simulink model "dft_bank_4"  (Simulink 7.8)
settings: Solver=ode45  StartTime=0.0  StopTime=1  RelTol=1e-3
values from neighbouring files (symbols this model uses):
  N = 2    [CFIR_1.m]    (also in TP_fdesign2.m = 128; cic_dezim1.m = ',num2str(N),')']); cic_dezim1_.m = ', num2str(N),' Gain = ',num2str(Hm.gain)]); cic_dezim2.m = ',num2str(N),')']))
  Ts = 1/fs    (= 6.25e-05)    [G722_1.m]    (also in adaptiv_2.m = 0.001; adaptiv_3.m = 0.001; adaptiv_4.m = 0.001; adaptiv_5.m = 0.001)
undefined symbols (not defined in the file or in its folder): Ksub, WN, WNt
libraries: dspsigops x1, dspobslib x1
settings Model: Creator=svenhoffmann  LastModifiedBy=josef  ExtModeAutoUpdateStatusClock=off
settings DataIOCC: SignalLoggingName=sigsOut
settings OptimizationCC: InitFltsAndDblsToZero=on
settings DebuggingCC: SaveWithParameterizedLinksMsg=none  SignalResolutionControl=TryResolveAllWithWarning  SolverPrmCheckMsg=none  MultiTaskDSMMsg=warning  MultiTaskCondExecSysMsg=none  FcnCallInpInsideContextMsg=Use local settings  StrictBusMsg=None
settings HardwareCC: TargetUnknown=on
settings RTWCC: IncludeERTFirstTime=on
settings GRTTargetCC: TargetFcnLib=ansi_tfl_tmw.mat

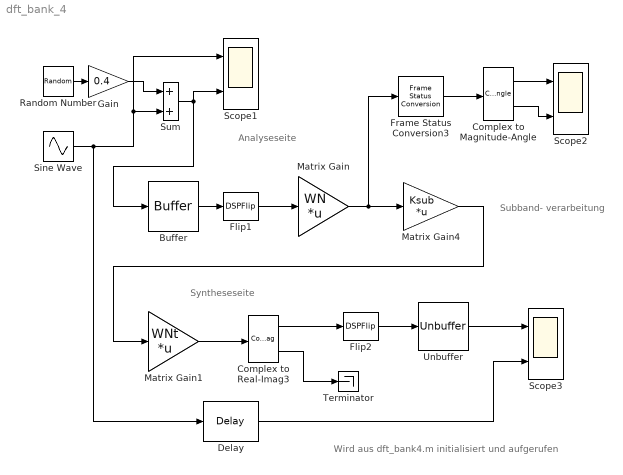
== system dft_bank_4 ==
  note: Analyseseite
  note: Syntheseseite
  note: Subband-
      | verarbeitung
  note: Wird aus dft_bank4.m initialisiert und aufgerufen
  Buffer : Buffer  N=N
  Complex to Magnitude-Angle : ComplexToMagnitudeAngle
  Complex to Real-Imag3 : ComplexToRealImag
  Delay : dspsigops/Delay  InputProcessing=Inherited (this choice will be removed - see release notes)  dly_unit=Samples  delay=10  ic_detail=off  dif_ic_for_ch=off  dif_ic_for_dly=off  ic=0  reset_popup=None
  Flip1 : DSPFlip
  Flip2 : DSPFlip
  Frame Status Conversion3 : dspobslib/Frame Status Conversion  growRefPort=off  outframe=Sample-based
  Gain : Gain  Gain=0.4  SaturateOnIntegerOverflow=on  OutDataTypeStr=Inherit: Same as input  ParamDataTypeStr=Inherit: Same as input
  Matrix Gain : Gain  Gain=WN  Multiplication=Matrix(K*u)  SaturateOnIntegerOverflow=on  OutDataTypeStr=Inherit: Same as input  ParamDataTypeStr=Inherit: Same as input
  Matrix Gain1 : Gain  Gain=WNt  Multiplication=Matrix(K*u)  SaturateOnIntegerOverflow=on  OutDataTypeStr=Inherit: Same as input  ParamDataTypeStr=Inherit: Same as input
  Matrix Gain4 : Gain  Gain=Ksub  Multiplication=Matrix(K*u)  SaturateOnIntegerOverflow=on  OutDataTypeStr=Inherit: Same as input  ParamDataTypeStr=Inherit: Same as input
  Random Number : RandomNumber  SampleTime=Ts
  Scope1 : Scope  NumInputPorts=2
      settings: TimeRange=1  YMin=-1~-1  YMax=1~1  SaveName=ScopeData2
  Scope2 : Scope  NumInputPorts=2
      settings: TimeRange=0.2  YMin=-8.32667e-17~-3  YMax=0.65~3.5
  Scope3 : Scope  NumInputPorts=2
      settings: TimeRange=0.199  YMin=-0.4~-1.25  YMax=0.4~1.25
  Sine Wave : Sin  Frequency=2*pi*100  SampleTime=Ts
  Sum : Sum  SaturateOnIntegerOverflow=on
  Terminator : Terminator
  Unbuffer : Unbuffer
  wires:
  Buffer/1 -> Flip1/1
  Flip1/1 -> Matrix Gain/1
  Matrix Gain/1 -> Frame Status Conversion3/1, Matrix Gain4/1
  Matrix Gain1/1 -> Complex to Real-Imag3/1
  Delay/1 -> Scope3/2
  Matrix Gain4/1 -> Matrix Gain1/1
  Complex to Magnitude-Angle/1 -> Scope2/1
  Complex to Magnitude-Angle/2 -> Scope2/2
  Frame Status Conversion3/1 -> Complex to Magnitude-Angle/1
  Flip2/1 -> Unbuffer/1
  Unbuffer/1 -> Scope3/1
  Random Number/1 -> Gain/1
  Sum/1 -> Buffer/1, Scope1/2
  Gain/1 -> Sum/1
  Sine Wave/1 -> Delay/1, Sum/2, Scope1/1
  Complex to Real-Imag3/1 -> Flip2/1
  Complex to Real-Imag3/2 -> Terminator/1
